simulink model "longitudinal_driver_2"  (R2024b)
settings: Solver=VariableStepAuto  StartTime=0.0  StopTime=10.0  RelTol=1e-3
undefined symbols (not defined in the file): car
libraries: simulink x8
settings Model: Creator=HP  LastModifiedBy=Loredana

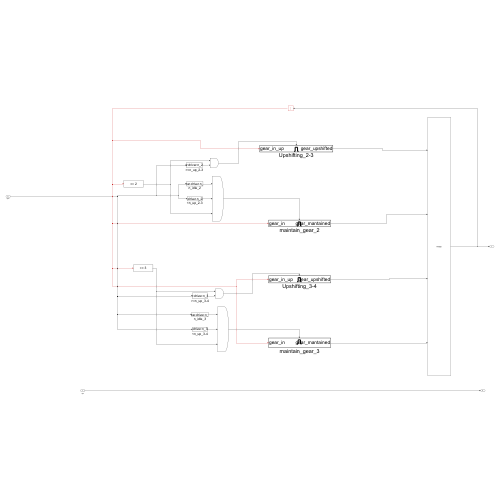
[thumbnail: Simulink's stored preview of the top-level diagram]
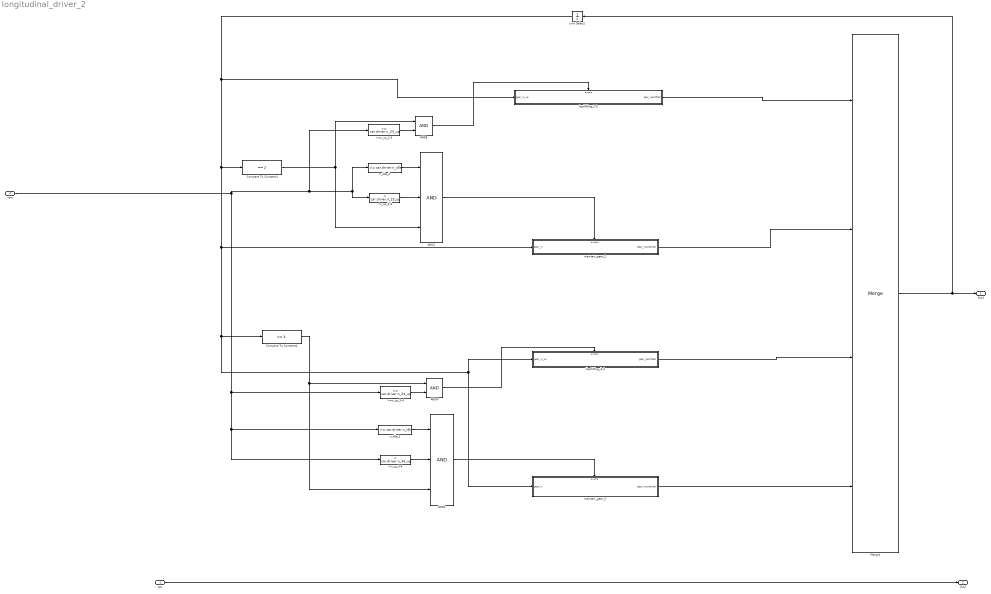
== system longitudinal_driver_2 ==
  tps : Inport
  rpm : Inport  Port=2
  <n_up_2-3 : simulink/Logic and Bit Operations/Compare To Constant  relop=<  const=car.driver.n_23_up  OutDataTypeStr=boolean
  <n_up_3-4 : simulink/Logic and Bit Operations/Compare To Constant  relop=<  const=car.driver.n_34_up  OutDataTypeStr=boolean
  >=n_up_2-3 : simulink/Logic and Bit Operations/Compare To Constant  relop=>=  const=car.driver.n_23_up  OutDataTypeStr=boolean
  >=n_up_3-4 : simulink/Logic and Bit Operations/Compare To Constant  relop=>=  const=car.driver.n_34_up  OutDataTypeStr=boolean
  AND1 : Logic  Inputs=3  IconShape=distinctive  AllPortsSameDT=off  OutDataTypeStr=boolean
  AND2 : Logic  Inputs=3  IconShape=distinctive  AllPortsSameDT=off  OutDataTypeStr=boolean
  AND4 : Logic  IconShape=distinctive  AllPortsSameDT=off  OutDataTypeStr=boolean
  AND8 : Logic  IconShape=distinctive  AllPortsSameDT=off  OutDataTypeStr=boolean
  Compare To Constant1 : simulink/Logic and Bit Operations/Compare To Constant  relop===  const=2  OutDataTypeStr=boolean
  Compare To Constant4 : simulink/Logic and Bit Operations/Compare To Constant  relop===  const=3  OutDataTypeStr=boolean
  Merge1 : Merge  Inputs=4
  Unit Delay2 : UnitDelay  InitialCondition=2  SampleTime=-1  HasFrameUpgradeWarning=on
  Upshifting_2-3 : Subsystem  TreatAsAtomicUnit=on
  Upshifting_3-4 : Subsystem  TreatAsAtomicUnit=on
  maintain_gear_2 : Subsystem  TreatAsAtomicUnit=on
  maintain_gear_3 : Subsystem  TreatAsAtomicUnit=on
  n_idle_2 : simulink/Logic and Bit Operations/Compare To Constant  relop=>=  const=car.driver.n_idle  OutDataTypeStr=boolean
  n_idle_3 : simulink/Logic and Bit Operations/Compare To Constant  relop=>=  const=car.driver.n_idle  OutDataTypeStr=boolean
  Out1 : Outport
  Out2 : Outport  Port=2
  wires:
  tps/1 -> Out2/1
  rpm/1 -> <n_up_2-3/1, n_idle_2/1, >=n_up_2-3/1, <n_up_3-4/1, n_idle_3/1, >=n_up_3-4/1
  maintain_gear_3/1(gear_mantained) -> Merge1/4
  n_idle_3/1 -> AND2/1
  Upshifting_2-3/1(gear_upshifted) -> Merge1/1
  AND2/1 -> maintain_gear_3/Enable
  Upshifting_3-4/1(gear_upshifted) -> Merge1/3
  AND1/1 -> maintain_gear_2/Enable
  AND8/1 -> Upshifting_2-3/Enable
  maintain_gear_2/1(gear_mantained) -> Merge1/2
  >=n_up_2-3/1 -> AND8/2
  Compare To Constant1/1 -> AND8/1, AND1/3
  <n_up_3-4/1 -> AND2/2
  <n_up_2-3/1 -> AND1/2
  n_idle_2/1 -> AND1/1
  AND4/1 -> Upshifting_3-4/Enable
  Merge1/1 -> Unit Delay2/1, Out1/1
  >=n_up_3-4/1 -> AND4/2
  Unit Delay2/1 -> Upshifting_2-3/1(gear_in_up), maintain_gear_3/1(gear_in), Upshifting_3-4/1(gear_in_up), Compare To Constant4/1, maintain_gear_2/1(gear_in), Compare To Constant1/1
  Compare To Constant4/1 -> AND2/3, AND4/1

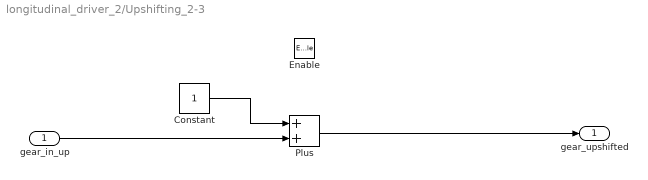
== system longitudinal_driver_2/Upshifting_2-3 ==
  gear_in_up : Inport
  Enable : EnablePort
  Constant : Constant
  Plus : Sum
  gear_upshifted : Outport
  wires:
  Plus/1 -> gear_upshifted/1
  Constant/1 -> Plus/1
  gear_in_up/1 -> Plus/2

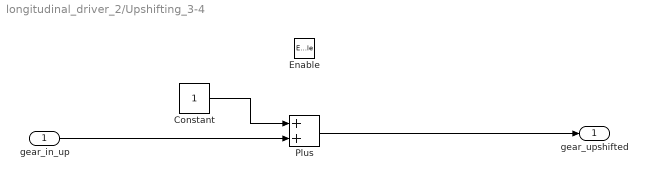
== system longitudinal_driver_2/Upshifting_3-4 ==
  gear_in_up : Inport
  Enable : EnablePort
  Constant : Constant
  Plus : Sum
  gear_upshifted : Outport
  wires:
  Plus/1 -> gear_upshifted/1
  Constant/1 -> Plus/1
  gear_in_up/1 -> Plus/2

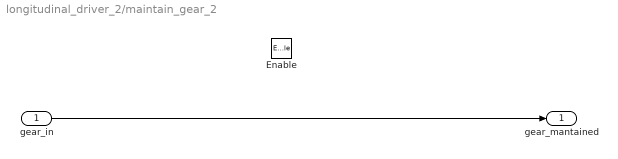
== system longitudinal_driver_2/maintain_gear_2 ==
  gear_in : Inport
  Enable : EnablePort
  gear_mantained : Outport
  wires:
  gear_in/1 -> gear_mantained/1

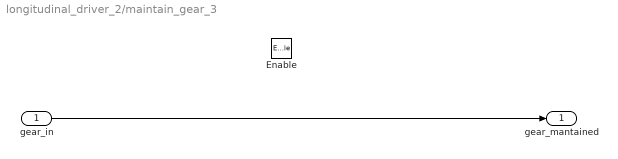
== system longitudinal_driver_2/maintain_gear_3 ==
  gear_in : Inport
  Enable : EnablePort
  gear_mantained : Outport
  wires:
  gear_in/1 -> gear_mantained/1
